simulink library "bcm"  (R2021b)
settings: Solver=VariableStepAuto  StartTime=0.0  StopTime=10.0  RelTol=1e-3
undefined symbols (not defined in the file or in its folder): ENUM_ANTITHEFT_ALARM, ENUM_ANTITHEFT_ARM, ENUM_ANTITHEFT_DISARM, ENUM_ANTITHEFT_WAIT, ENUM_GEARPOSNTOCAN_P, ENUM_PDKEYRAWLULOCK_INUNLOCK, ENUM_PDKEYRAWPS_INPS, ENUM_POWERSTA_READY, ENUM_POWERSTA_STANDBY, FALSE, KBCM_ALMBrightnessDark_enum, KBCM_AmbBlue_enum, KBCM_AmbBreathT_K, KBCM_AmbBreathTOut_K, KBCM_AmbGreen_enum, KBCM_AmbLightUser_enum, KBCM_AmbPreset_enum, KBCM_AmbRed_enum, KBCM_Antitheft_enum_ovrdflg, KBCM_Antitheft_enum_ovrdval, KBCM_APMDoorCtrlSta_flg_ovrdflg, KBCM_APMDoorCtrlSta_flg_ovrdval, KBCM_DelayTSW_flg, KBCM_DiagFLTC_mA, KBCM_DiagFMHT_s, KBCM_DiagFRTC_mA, KBCM_DiagRLTC_mA, KBCM_DiagRRTC_mA, KBCM_DrAPMRetryTimes_cnt, KBCM_DrOpenWdwOT_s, KBCM_DrOpenWdwReady_s, KBCM_ESSOffT_ms, KBCM_ESSOnT_ms, KBCM_IVIRstHoldT_ms, KBCM_IVIRstTriggerT_ms, KBCM_ONDelayT_ms, KBCM_ReDetectT_K, KBCM_RmLampKeep_min, KBCM_RmLpKeyInT_s, KBCM_RmLpKeyMissT_s, KBCM_SlpDebounceTime_s, KBCM_SPTGDetectT_sec, KBCM_SPTGLeave_flg, KBCM_SPTGLeftBound_cm, KBCM_SPTGLeftBoundOut_cm, KBCM_SPTGLowerBound_cm, KBCM_SPTGLowerBoundOut_cm, KBCM_SPTGRightBound_cm, KBCM_SPTGRightBoundOut_cm, KBCM_SPTGTOut_K, KBCM_SPTGUpperBound_cm, KBCM_SPTGUpperBoundOut_cm, KBCM_SPTGWaitDKC_sec, KBCM_USSDis_cm, KBCM_USSFilterT_K, KBCM_WaitAPMPwr_K, KBCM_WdwManualDetT_s, MIN2SEC, TRUE, XX2KXX
libraries: simulink x41, $bdroot x3, hcu_lib x2
(part 3 of 6)

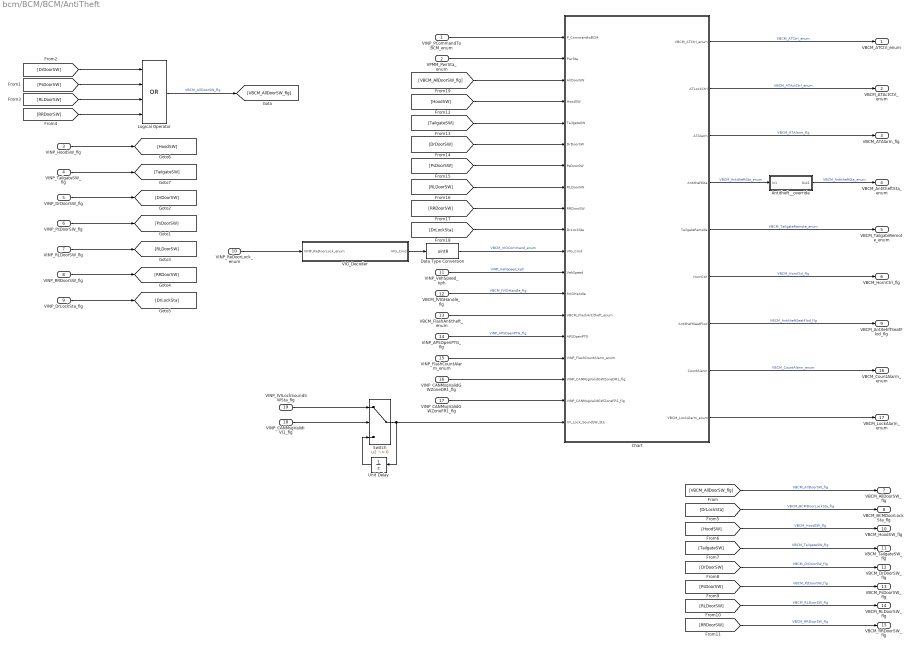
== system bcm/BCM/BCM/AntiTheft ==
  VINP_PCommandToBCM_enum : Inport
  VPMM_PwrSta_enum : Inport  Port=2
  VINP_HoodSW_flg : Inport  Port=3
  VINP_TailgateSW_flg : Inport  Port=4
  VINP_DrDoorSW_flg : Inport  Port=5
  VINP_PsDoorSW_flg : Inport  Port=6
  VINP_RLDoorSW_flg : Inport  Port=7
  VINP_RRDoorSW_flg : Inport  Port=8
  VINP_DrLockSta_flg : Inport  Port=9
  VINP_ReDoorLock_enum : Inport  Port=10
  VINP_VehSpeed_kph : Inport  Port=11
  VBCM_fVIGHandle_flg : Inport  Port=12
  VBCM_FlashAntitheft_enum : Inport  Port=13
  VINP_APSOpenPTG_flg : Inport  Port=14
  VINP_FlashCountAlarm_enum : Inport  Port=15
  VINP_CANMsgValidGWZoneDR1_flg : Inport  Port=16
  VINP_CANMsgValidGWZoneFR1_flg : Inport  Port=17
  VINP_CANMsgValidIVI1_flg : Inport  Port=18
  VINP_IVILockSoundSWSta_flg : Inport  Port=19
  Antitheft__override : Subsystem
  Chart : Stateflow chart  TreatAsAtomicUnit=on
      settings: PortSchema="{\"entries\":[{\"content\":{\"sides\":[{\"content\":{\"connectorIds\":[\"In1\",\"In2\",\"In3\",\"In4\",\"In5\",\"In6\",\"In7\",\"In8\",\"In9\",\"In10\",\"In11\",\"In12\",\"In13\",\"In14\",\"In15\",\"In16\",\"In17\",\"In18\",\"In19\"]},\"type\":\"ConnectorPlacement.EquallySpacedRectSide\",\"uuid\":\"1a74f1bb-1441-4b1e-a72b-a3afd3d564cb\"},{\"content\":{\"connectorIds\":[\"Out8\",\"Out1\",\"Out2\",\"Out3\",\"Out4\",\"Out5\",\"Out6\",\"Out7\",\"Out9\"],\"side\":\"RIGHT\"},\"type\":\"ConnectorPlacement.EquallySpacedRectSide\",\"uuid\":\"1f80d4d2-2ca7-43bd-b54c-63979ded17e1\"},{\"content\":{\"side\":\"TOP\"},\"type\":\"ConnectorPlacement.EquallySpacedRectSide\",\"uuid\":\"a2ec125f-5165-4db1-a6b4-591b84a723ff\"}]},\"type\":\"ConnectorPlacement.EquallySpacedConnector\",\"uuid\":\"5ff7fbe4-0c2a-42b5-89b8-60500b2b9a9a\"}],\"packageUris\":[\"http://schema.mathworks.com/mf0/Connector/R2020b\"],\"version\":\"1.0\"}"
  Data Type Conversion : DataTypeConversion  OutDataTypeStr=uint8
  Logical Operator : Logic  Operator=OR  Inputs=4  AllPortsSameDT=off  OutDataTypeStr=boolean
  Switch : Switch  Criteria=u2 ~= 0
  Unit Delay : UnitDelay  SampleTime=-1  HasFrameUpgradeWarning=on
  VIG_Decoder : MATLAB Function  TreatAsAtomicUnit=on
  VBCM_ATCtrl_enum : Outport
  VBCM_ATActCtrl_enum : Outport  Port=2
  VBCM_ATAlarm_flg : Outport  Port=3
  VBCM_AntitheftSta_enum : Outport  Port=4
  VBCM_TailgateRemote_enum : Outport  Port=5
  VBCM_HornCtrl_flg : Outport  Port=6
  VBCM_AllDoorSW_flg : Outport  Port=7
  VBCM_BCMDoorLockSta_flg : Outport  Port=8
  VBCM_AntitehftSeatFlod_flg : Outport  Port=9
  VBCM_HoodSW_flg : Outport  Port=10
  VBCM_TailgateSW_flg : Outport  Port=11
  VBCM_DrDoorSW_flg : Outport  Port=12
  VBCM_PsDoorSW_flg : Outport  Port=13
  VBCM_RLDoorSW_flg : Outport  Port=14
  VBCM_RRDoorSW_flg : Outport  Port=15
  VBCM_CountAlarm_enum : Outport  Port=16
  VBCM_LockAlarm_enum : Outport  Port=17
  wires:
  VBCM_fVIGHandle_flg/1 -> Chart/13(fVIGHandle)  "VBCM_fVIGHandle_flg"
  VINP_RRDoorSW_flg/1 -> [RRDoorSW]
  VINP_ReDoorLock_enum/1 -> VIG_Decoder/1(VINP_ReDoorLock_enum)
  Chart/1(ATLockCtrl) -> VBCM_ATActCtrl_enum/1  "VBCM_ATActCtrl_enum"
  Chart/8(VBCM_ATCtrl_enum) -> VBCM_ATCtrl_enum/1  "VBCM_ATCtrl_enum"
  VINP_PCommandToBCM_enum/1 -> Chart/1(P_CommandtoBCM)
  VINP_RLDoorSW_flg/1 -> [RLDoorSW]
  Chart/2(ATAlarm) -> VBCM_ATAlarm_flg/1  "VBCM_ATAlarm_flg"
  VINP_PsDoorSW_flg/1 -> [PsDoorSW]
  VINP_VehSpeed_kph/1 -> Chart/12(VehSpeed)  "VINP_VehSpeed_kph"
  Logical Operator/1 -> [VBCM_AllDoorSW_flg]  "VBCM_AllDoorSW_flg"
  VINP_DrDoorSW_flg/1 -> [DrDoorSW]
  VINP_HoodSW_flg/1 -> [HoodSW]
  VIG_Decoder/1(VIG_Cmd) -> Data Type Conversion/1
  Data Type Conversion/1 -> Chart/11(VIG_Cmd)  "VBCM_VIGCommand_enum"
  [VBCM_AllDoorSW_flg] -> VBCM_AllDoorSW_flg/1  "VBCM_AllDoorSW_flg"
  Chart/3(AntitheftSta) -> Antitheft__override/1(In1)  "VBCM_AntitheftSta_enum"
  Chart/4(TailgateRemote) -> VBCM_TailgateRemote_enum/1  "VBCM_TailgateRemote_enum"
  Chart/5(HornCtrl) -> VBCM_HornCtrl_flg/1  "VBCM_HornCtrl_flg"
  Chart/6(AntitheftSeatFlod) -> VBCM_AntitehftSeatFlod_flg/1  "VBCM_AntitheftSeatFlod_flg"
  Antitheft__override/1(Out1) -> VBCM_AntitheftSta_enum/1  "VBCM_AntitheftSta_enum"
  VINP_APSOpenPTG_flg/1 -> Chart/15(APSOpenPTG)  "VINP_APSOpenPTG_flg"
  VINP_TailgateSW_flg/1 -> [TailgateSW]
  [DrDoorSW] -> Logical Operator/1
  [PsDoorSW] -> Logical Operator/2
  [RLDoorSW] -> Logical Operator/3
  [RRDoorSW] -> Logical Operator/4
  VINP_DrLockSta_flg/1 -> [DrLockSta]
  [DrLockSta] -> VBCM_BCMDoorLockSta_flg/1  "VBCM_BCMDoorLockSta_flg"
  [HoodSW] -> VBCM_HoodSW_flg/1  "VBCM_HoodSW_flg"
  [TailgateSW] -> VBCM_TailgateSW_flg/1  "VBCM_TailgateSW_flg"
  [DrDoorSW] -> VBCM_DrDoorSW_flg/1  "VBCM_DrDoorSW_flg"
  [PsDoorSW] -> VBCM_PsDoorSW_flg/1  "VBCM_PsDoorSW_flg"
  [RLDoorSW] -> VBCM_RLDoorSW_flg/1  "VBCM_RLDoorSW_flg"
  [RRDoorSW] -> VBCM_RRDoorSW_flg/1  "VBCM_RRDoorSW_flg"
  VPMM_PwrSta_enum/1 -> Chart/2(PwrSta)
  VBCM_FlashAntitheft_enum/1 -> Chart/14(VBCM_FlashAntitheft_enum)
  [DrDoorSW] -> Chart/6(DrDoorSW)
  [TailgateSW] -> Chart/5(TailgateSW)
  [PsDoorSW] -> Chart/7(PsDoorSW)
  [HoodSW] -> Chart/4(HoodSW)
  [RRDoorSW] -> Chart/9(RRDoorSW)
  [RLDoorSW] -> Chart/8(RLDoorSW)
  [DrLockSta] -> Chart/10(DrLockSta)
  [VBCM_AllDoorSW_flg] -> Chart/3(AllDoorSW)
  VINP_FlashCountAlarm_enum/1 -> Chart/16(VINP_FlashCountAlarm_enum)
  VINP_CANMsgValidGWZoneDR1_flg/1 -> Chart/17(VINP_CANMsgValidGWZoneDR1_flg)
  VINP_CANMsgValidGWZoneFR1_flg/1 -> Chart/18(VINP_CANMsgValidGWZoneFR1_flg)
  Chart/7(CountAlarm) -> VBCM_CountAlarm_enum/1  "VBCM_CountAlarm_enum"
  Chart/9(VBCM_LockAlarm_enum) -> VBCM_LockAlarm_enum/1
  VINP_CANMsgValidIVI1_flg/1 -> Switch/2
  Unit Delay/1 -> Switch/3
  Switch/1 -> Chart/19(IVI_Lock_SoundSW_Sta), Unit Delay/1
  VINP_IVILockSoundSWSta_flg/1 -> Switch/1

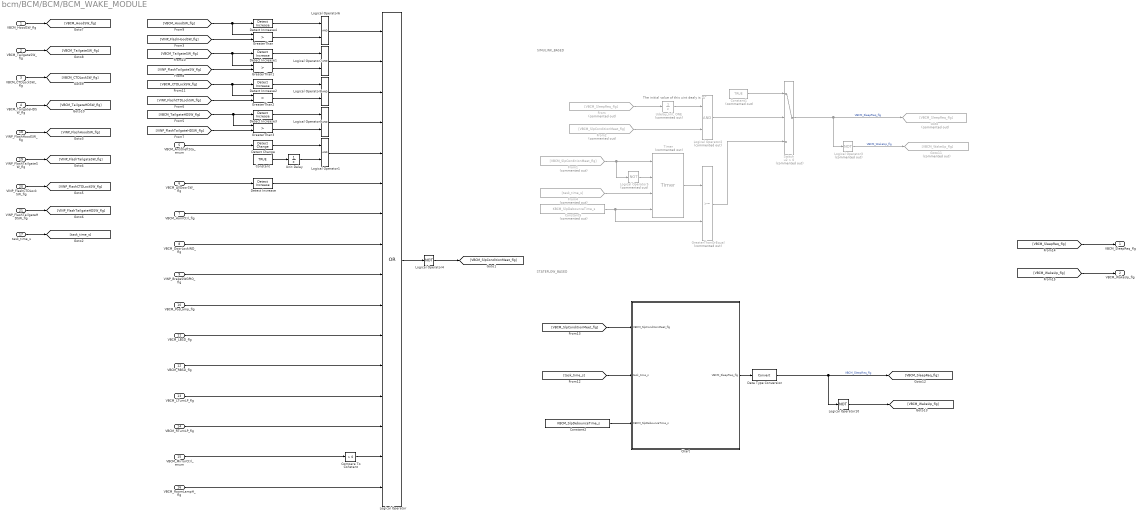
== system bcm/BCM/BCM/BCM_WAKE_MODULE ==
  note: SIMULINK_BASED
  note: STATEFLOW_BASED
  note: The initial value of this uint dealy is "1"
  VBCM_HoodSW_flg : Inport
  VBCM_TailgateSW_flg : Inport  Port=2
  VBCM_CTDLockSW_flg : Inport  Port=3
  VBCM_TailgateHDSW_flg : Inport  Port=4
  VBCM_AntitheftSta_enum : Inport  Port=5
  VBCM_AllDoorSW_flg : Inport  Port=6
  VBCM_HornCtrl_flg : Inport  Port=7
  VBCM_DoorLockIND_flg : Inport  Port=8
  VINP_BrakeSWGPIO_flg : Inport  Port=9
  VBCM_PosLamp_flg : Inport  Port=10
  VBCM_LBSD_flg : Inport  Port=11
  VBCM_RBSD_flg : Inport  Port=12
  VBCM_LTurnLP_flg : Inport  Port=13
  VBCM_RTurnLP_flg : Inport  Port=14
  VBCM_MirrorCtrl_enum : Inport  Port=15
  VBCM_RoomLampH_flg : Inport  Port=16
  task_time_s : Inport  Port=17
  VINP_FlashHoodSW_flg : Inport  Port=18
  VINP_FlashTailgateSW_flg : Inport  Port=19
  VINP_FlashCTDLockSW_flg : Inport  Port=20
  VINP_FlashTailgateHDSW_flg : Inport  Port=21
  Chart : Stateflow chart  TreatAsAtomicUnit=on
  Compare To Constant : simulink/Logic and Bit Operations/Compare To Constant  relop=>  const=0  OutDataTypeStr=boolean
  Constant : Constant  Value=TRUE
  Constant1 : Constant  Commented=on  Value=TRUE
  Constant2 : Constant  Value=KBCM_SlpDebounceTime_s
  Constant5 : Constant  Commented=on  Value=KBCM_SlpDebounceTime_s
  Data Type Conversion : DataTypeConversion
  Detect Change : simulink/Logic and Bit Operations/Detect Change  vinit=0  OutDataTypeStr=boolean
  Detect Increase{,1..4} (5 alike) : simulink/Logic and Bit Operations/Detect Increase  vinit=0.0  OutDataTypeStr=boolean
  From : From  Commented=on  GotoTag=VBCM_SleepReq_flg
  From1 : From  Commented=on  GotoTag=VBCM_SlpConditionMeet_flg
  From2 : From  Commented=on  GotoTag=VBCM_SlpConditionMeet_flg
  From4 : From  Commented=on  GotoTag=task_time_s
  Goto : Goto  Commented=on  GotoTag=VBCM_SleepReq_flg
  Goto11 : Goto  Commented=on  GotoTag=VBCM_WakeUp_flg
  GreaterThan{,1..3} (4 alike) : RelationalOperator  Operator=>  OutDataTypeStr=boolean  RndMeth=Simplest
  GreaterThanOrEqual : RelationalOperator  Commented=on  OutDataTypeStr=boolean  RndMeth=Simplest
  Logical Operator : Logic  Operator=OR  Inputs=16  AllPortsSameDT=off  OutDataTypeStr=boolean
  Logical Operator{1,6..9} (5 alike) : Logic  AllPortsSameDT=off  OutDataTypeStr=boolean
  Logical Operator10 : Logic  Operator=NOT  AllPortsSameDT=off  OutDataTypeStr=boolean
  Logical Operator2 : Logic  Commented=on  AllPortsSameDT=off  OutDataTypeStr=boolean
  Logical Operator3 : Logic  Commented=on  Operator=NOT  AllPortsSameDT=off  OutDataTypeStr=boolean
  Logical Operator4 : Logic  Operator=NOT  AllPortsSameDT=off  OutDataTypeStr=boolean
  Logical Operator5 : Logic  Commented=on  Operator=NOT  AllPortsSameDT=off  OutDataTypeStr=boolean
  Switch : Switch  Commented=on  Criteria=u2 > Threshold
  Timer : hcu_lib/Basic_Blocks/Timer  Commented=on
  Udelay_Init_ONE : UnitDelay  Commented=on  InitialCondition=1  SampleTime=-1  HasFrameUpgradeWarning=on
  Unit Delay : UnitDelay  SampleTime=-1  HasFrameUpgradeWarning=on
  VBCM_SleepReq_flg : Outport
  VBCM_WakeUp_flg : Outport  Port=2
  wires:
  VBCM_DoorLockIND_flg/1 -> Logical Operator/8
  VBCM_LBSD_flg/1 -> Logical Operator/11
  VBCM_RoomLampH_flg/1 -> Logical Operator/16
  VBCM_RBSD_flg/1 -> Logical Operator/12
  VBCM_HornCtrl_flg/1 -> Logical Operator/7
  VBCM_AllDoorSW_flg/1 -> Detect Increase/1
  VBCM_RTurnLP_flg/1 -> Logical Operator/14
  Compare To Constant/1 -> Logical Operator/15
  VBCM_PosLamp_flg/1 -> Logical Operator/10
  VINP_BrakeSWGPIO_flg/1 -> Logical Operator/9
  VBCM_MirrorCtrl_enum/1 -> Compare To Constant/1
  VBCM_LTurnLP_flg/1 -> Logical Operator/13
  Detect Change/1 -> Logical Operator1/1
  VBCM_AntitheftSta_enum/1 -> Detect Change/1
  Constant5/1 -> GreaterThanOrEqual/2, Timer/4
  Timer/1 -> GreaterThanOrEqual/1
  Logical Operator/1 -> Logical Operator4/1
  Logical Operator1/1 -> Logical Operator/5
  Unit Delay/1 -> Logical Operator1/2
  Constant/1 -> Unit Delay/1
  Logical Operator4/1 -> [VBCM_SlpConditionMeet_flg]
  Switch/1 -> Logical Operator3/1, Goto/1  "VBCM_SleepReq_flg"
  Logical Operator2/1 -> Switch/2
  Constant1/1 -> Switch/1
  From/1 -> Udelay_Init_ONE/1
  GreaterThanOrEqual/1 -> Switch/3
  Udelay_Init_ONE/1 -> Logical Operator2/1
  Logical Operator5/1 -> Timer/2
  From2/1 -> Logical Operator2/2
  From1/1 -> Logical Operator5/1, Timer/1
  task_time_s/1 -> [task_time_s]
  From4/1 -> Timer/3
  VBCM_HoodSW_flg/1 -> [VBCM_HoodSW_flg]
  [VINP_FlashHoodSW_flg] -> GreaterThan/2
  GreaterThan/1 -> Logical Operator6/2
  Logical Operator6/1 -> Logical Operator/1
  [VBCM_HoodSW_flg] -> GreaterThan/1, Detect Increase4/1
  Detect Increase4/1 -> Logical Operator6/1
  VBCM_TailgateSW_flg/1 -> [VBCM_TailgateSW_flg]
  [VBCM_CTDLockSW_flg] -> Detect Increase2/1, GreaterThan2/1
  Detect Increase2/1 -> Logical Operator8/1
  GreaterThan2/1 -> Logical Operator8/2
  Logical Operator8/1 -> Logical Operator/3
  [VINP_FlashCTDLockSW_flg] -> GreaterThan2/2
  VBCM_CTDLockSW_flg/1 -> [VBCM_CTDLockSW_flg]
  [VBCM_TailgateHDSW_flg] -> Detect Increase3/1, GreaterThan3/1
  Detect Increase3/1 -> Logical Operator9/1
  [VINP_FlashTailgateHDSW_flg] -> GreaterThan3/2
  GreaterThan3/1 -> Logical Operator9/2
  VBCM_TailgateHDSW_flg/1 -> [VBCM_TailgateHDSW_flg]
  GreaterThan1/1 -> Logical Operator7/2
  Logical Operator7/1 -> Logical Operator/2
  [VINP_FlashTailgateSW_flg] -> GreaterThan1/2
  [VBCM_TailgateSW_flg] -> GreaterThan1/1, Detect Increase1/1
  Detect Increase1/1 -> Logical Operator7/1
  Logical Operator9/1 -> Logical Operator/4
  VINP_FlashHoodSW_flg/1 -> [VINP_FlashHoodSW_flg]
  VINP_FlashTailgateSW_flg/1 -> [VINP_FlashTailgateSW_flg]
  VINP_FlashCTDLockSW_flg/1 -> [VINP_FlashCTDLockSW_flg]
  VINP_FlashTailgateHDSW_flg/1 -> [VINP_FlashTailgateHDSW_flg]
  [task_time_s] -> Chart/2(task_time_s)
  Constant2/1 -> Chart/3(KBCM_SlpDebounceTime_s)
  [VBCM_SlpConditionMeet_flg] -> Chart/1(VBCM_SlpConditionMeet_flg)
  Logical Operator3/1 -> Goto11/1  "VBCM_WakeUp_flg"
  [VBCM_SleepReq_flg] -> VBCM_SleepReq_flg/1
  [VBCM_WakeUp_flg] -> VBCM_WakeUp_flg/1
  Logical Operator10/1 -> [VBCM_WakeUp_flg]
  Data Type Conversion/1 -> Logical Operator10/1, [VBCM_SleepReq_flg]  "VBCM_SleepReq_flg"
  Chart/1(VBCM_SleepReq_flg) -> Data Type Conversion/1
  Detect Increase/1 -> Logical Operator/6

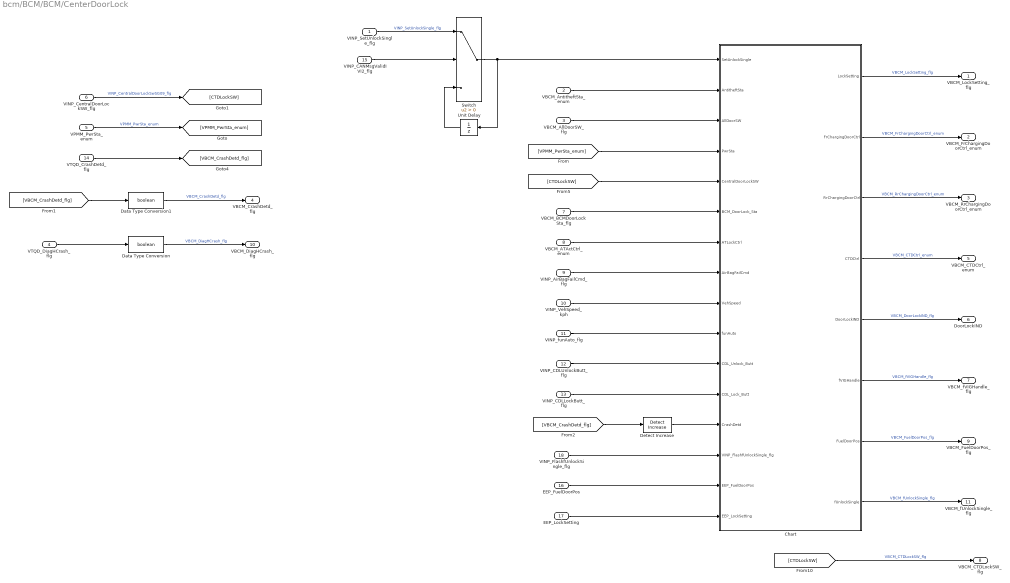
== system bcm/BCM/BCM/CenterDoorLock ==
  VINP_SetUnlockSingle_flg : Inport
  VBCM_AntitheftSta_enum : Inport  Port=2
  VBCM_AllDoorSW_flg : Inport  Port=3  OutDataTypeStr=boolean
  VTQD_DiagHCrash_flg : Inport  Port=4
  VPMM_PwrSta_enum : Inport  Port=5
  VINP_CentralDoorLockSW_flg : Inport  Port=6
  VBCM_BCMDoorLockSta_flg : Inport  Port=7
  VBCM_ATActCtrl_enum : Inport  Port=8
  VINP_AirBagFailCmd_flg : Inport  Port=9
  VINP_VehSpeed_kph : Inport  Port=10
  VINP_funAuto_flg : Inport  Port=11
  VINP_CDLUnlockButt_flg : Inport  Port=12  OutDataTypeStr=boolean
  VINP_CDLLockButt_flg : Inport  Port=13  OutDataTypeStr=boolean
  VTQD_CrashDetd_flg : Inport  Port=14
  VINP_CANMsgValidIVI2_flg : Inport  Port=15
  EEP_FuelDoorPos : Inport  Port=16
  EEP_LockSetting : Inport  Port=17
  VINP_FlashfUnlockSingle_flg : Inport  Port=18
  Chart : Stateflow chart  TreatAsAtomicUnit=on
  Data Type Conversion : DataTypeConversion  OutDataTypeStr=boolean
  Data Type Conversion1 : DataTypeConversion  OutDataTypeStr=boolean
  Detect Increase : simulink/Logic and Bit Operations/Detect Increase  vinit=0.0  OutDataTypeStr=boolean
  Switch : Switch  Criteria=u2 > Threshold
  Unit Delay : UnitDelay  SampleTime=-1  HasFrameUpgradeWarning=on
  VBCM_LockSetting_flg : Outport
  VBCM_FrChargingDoorCtrl_enum : Outport  Port=2
  VBCM_RrChargingDoorCtrl_enum : Outport  Port=3
  VBCM_CrashDetd_flg : Outport  Port=4
  VBCM_CTDCtrl_enum : Outport  Port=5
  DoorLockIND : Outport  Port=6
  VBCM_fVIGHandle_flg : Outport  Port=7
  VBCM_CTDLockSW_flg : Outport  Port=8
  VBCM_FuelDoorPos_flg : Outport  Port=9
  VBCM_DiagHCrash_flg : Outport  Port=10
  VBCM_fUnlockSingle_flg : Outport  Port=11
  wires:
  VBCM_AntitheftSta_enum/1 -> Chart/2(AntitheftSta)
  VINP_CDLUnlockButt_flg/1 -> Chart/11(CDL_Unlock_Butt)
  Chart/6(fVIGHandle) -> VBCM_fVIGHandle_flg/1  "VBCM_fVIGHandle_flg"
  Chart/1(LockSetting) -> VBCM_LockSetting_flg/1  "VBCM_LockSetting_flg"
  VINP_funAuto_flg/1 -> Chart/10(funAuto)
  VINP_VehSpeed_kph/1 -> Chart/9(VehSpeed)
  VINP_AirBagFailCmd_flg/1 -> Chart/8(AirBagFailCmd)
  VBCM_ATActCtrl_enum/1 -> Chart/7(ATLockCtrl)
  Chart/5(DoorLockIND) -> DoorLockIND/1  "VBCM_DoorLockIND_flg"
  VBCM_AllDoorSW_flg/1 -> Chart/3(AllDoorSW)
  Chart/2(FrChargingDoorCtrl) -> VBCM_FrChargingDoorCtrl_enum/1  "VBCM_FrChargingDoorCtrl_enum"
  Chart/3(RrChargingDoorCtrl) -> VBCM_RrChargingDoorCtrl_enum/1  "VBCM_RrChargingDoorCtrl_enum"
  VBCM_BCMDoorLockSta_flg/1 -> Chart/6(BCM_DoorLock_Sta)
  VINP_SetUnlockSingle_flg/1 -> Switch/1  "VINP_SetUnlockSingle_flg"
  Chart/4(CTDCtrl) -> VBCM_CTDCtrl_enum/1  "VBCM_CTDCtrl_enum"
  VINP_CDLLockButt_flg/1 -> Chart/12(CDL_Lock_Butt)
  [CTDLockSW] -> VBCM_CTDLockSW_flg/1  "VBCM_CTDLockSW_flg"
  Unit Delay/1 -> Switch/3
  Switch/1 -> Chart/1(SetUnlockSingle), Unit Delay/1
  VINP_CANMsgValidIVI2_flg/1 -> Switch/2
  VPMM_PwrSta_enum/1 -> [VPMM_PwrSta_enum]  "VPMM_PwrSta_enum"
  [VPMM_PwrSta_enum] -> Chart/4(PwrSta)
  VTQD_CrashDetd_flg/1 -> [VBCM_CrashDetd_flg]
  VINP_CentralDoorLockSW_flg/1 -> [CTDLockSW]  "VINP_CentralDoorLockSwSG09_flg"
  [CTDLockSW] -> Chart/5(CentralDoorLockSW)
  Detect Increase/1 -> Chart/13(CrashDetd)
  [VBCM_CrashDetd_flg] -> Detect Increase/1
  Data Type Conversion/1 -> VBCM_DiagHCrash_flg/1  "VBCM_DiagHCrash_flg"
  Data Type Conversion1/1 -> VBCM_CrashDetd_flg/1  "VBCM_CrashDetd_flg"
  VTQD_DiagHCrash_flg/1 -> Data Type Conversion/1
  [VBCM_CrashDetd_flg] -> Data Type Conversion1/1
  EEP_FuelDoorPos/1 -> Chart/15(EEP_FuelDoorPos)
  Chart/7(FuelDoorPos) -> VBCM_FuelDoorPos_flg/1  "VBCM_FuelDoorPos_flg"
  EEP_LockSetting/1 -> Chart/16(EEP_LockSetting)
  VINP_FlashfUnlockSingle_flg/1 -> Chart/14(VINP_FlashfUnlockSingle_flg)
  Chart/8(fUnlockSingle) -> VBCM_fUnlockSingle_flg/1  "VBCM_fUnlockSingle_flg"

== system bcm/BCM/BCM/Dimmer ==
  VINP_MFRDNBrightReq_pct : Inport
  VINP_IVIStatus_flg : Inport  Port=2
  VINP_IVINightModeSta_flg : Inport  Port=3
  VBCM_PosLamp_flag : Inport  Port=4
  VINP_CANMsgValidIVI2_flg : Inport  Port=5
  EEP_MFRDNBrightReq : Inport  Port=6
  BCMInitial : Inport  Port=7
  Chart : Stateflow chart  TreatAsAtomicUnit=on
      settings: PortSchema="{\"entries\":[{\"content\":{\"sides\":[{\"content\":{\"connectorIds\":[\"In4\",\"In1\",\"In2\",\"In3\"]},\"type\":\"ConnectorPlacement.EquallySpacedRectSide\",\"uuid\":\"076f305a-8f7e-4e65-8c9e-aa6699a69b21\"},{\"content\":{\"connectorIds\":[\"Out1\",\"Out2\"],\"side\":\"RIGHT\"},\"type\":\"ConnectorPlacement.EquallySpacedRectSide\",\"uuid\":\"bf947e95-3d60-4849-99c4-9fb941c8d282\"},{\"content\":{\"side\":\"TOP\"},\"type\":\"ConnectorPlacement.EquallySpacedRectSide\",\"uuid\":\"13c4efb7-da15-49ea-8253-a9d27aa3456c\"}]},\"type\":\"ConnectorPlacement.EquallySpacedConnector\",\"uuid\":\"7282b60f-551e-46a0-a3a5-beda89adbd0d\"}],\"packageUris\":[\"http://schema.mathworks.com/mf0/Connector/R2020b\"],\"version\":\"1.0\"}"
  Data Type Conversion1 : DataTypeConversion
  Switch1 : Switch  Criteria=u2 > Threshold
  Switch2 : Switch  Criteria=u2 > Threshold
  Switch3 : Switch  Criteria=u2 > Threshold
  Unit Delay : UnitDelay  SampleTime=-1  HasFrameUpgradeWarning=on
  Unit Delay1 : UnitDelay  SampleTime=-1  HasFrameUpgradeWarning=on
  VBCM_Dimmer_pct : Outport
  VBCM_DimmerEN_flg : Outport  Port=2
  VBCM_MFRDNBrightReq_pct : Outport  Port=3
  wires:
  VBCM_PosLamp_flag/1 -> Chart/3(PLamp)
  Chart/1(Dimmer) -> VBCM_Dimmer_pct/1  "VBCM_Dimmer_pct"
  VINP_IVIStatus_flg/1 -> Chart/1(IVI_Status)
  Chart/2(DimmerEN) -> VBCM_DimmerEN_flg/1  "VBCM_DimmerEN_flg"
  VINP_IVINightModeSta_flg/1 -> Switch1/1  "VINP_IVINightModeSta_flg"
  VINP_CANMsgValidIVI2_flg/1 -> Switch2/2, Switch1/2  "VINP_CANMsgValidIVI2_flg"
  Switch1/1 -> Unit Delay1/1, Chart/2(IVI_Night_Mode_Sta)
  Unit Delay1/1 -> Switch1/3
  BCMInitial/1 -> Switch3/2
  EEP_MFRDNBrightReq/1 -> Switch3/3
  Switch3/1 -> Data Type Conversion1/1, Unit Delay/1
  Switch2/1 -> Switch3/1
  Unit Delay/1 -> Switch2/3
  VINP_MFRDNBrightReq_pct/1 -> Switch2/1
  Data Type Conversion1/1 -> VBCM_MFRDNBrightReq_pct/1, Chart/4(MFRD_N_Bright_Req)  "VBCM_MFRDNBrightReq_pct"

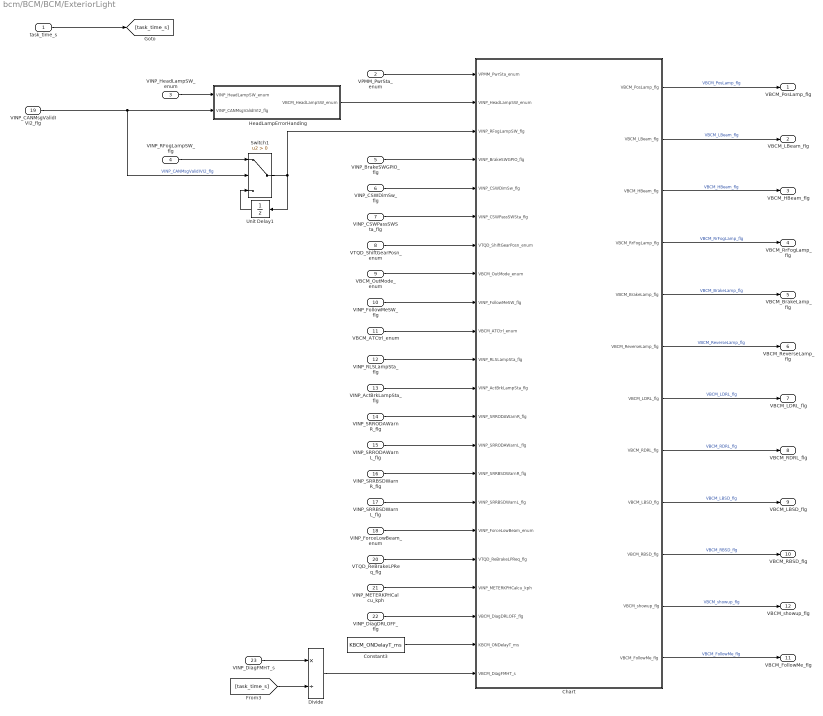
== system bcm/BCM/BCM/ExteriorLight ==
  task_time_s : Inport
  VPMM_PwrSta_enum : Inport  Port=2
  VINP_HeadLampSW_enum : Inport  Port=3
  VINP_RFogLampSW_flg : Inport  Port=4
  VINP_BrakeSWGPIO_flg : Inport  Port=5
  VINP_CSWDimSw_flg : Inport  Port=6
  VINP_CSWPassSWSta_flg : Inport  Port=7
  VTQD_ShiftGearPosn_enum : Inport  Port=8
  VBCM_OutMode_enum : Inport  Port=9
  VINP_FollowMeSW_flg : Inport  Port=10
  VBCM_ATCtrl_enum : Inport  Port=11
  VINP_RLSLampSta_flg : Inport  Port=12
  VINP_ActBrkLampSta_flg : Inport  Port=13
  VINP_SRRODAWarnR_flg : Inport  Port=14
  VINP_SRRODAWarnL_flg : Inport  Port=15
  VINP_SRRBSDWarnR_flg : Inport  Port=16
  VINP_SRRBSDWarnL_flg : Inport  Port=17
  VINP_ForceLowBeam_enum : Inport  Port=18
  VINP_CANMsgValidIVI2_flg : Inport  Port=19
  VTQD_ReBrakeLPReq_flg : Inport  Port=20
  VINP_METERKPHCalcu_kph : Inport  Port=21
  VINP_DiagDRLOFF_flg : Inport  Port=22
  VINP_DiagFMHT_s : Inport  Port=23
  Chart : Stateflow chart  TreatAsAtomicUnit=on
      settings: PortSchema="{\"entries\":[{\"content\":{\"sides\":[{\"content\":{\"connectorIds\":[\"In1\",\"In2\",\"In3\",\"In4\",\"In5\",\"In6\",\"In7\",\"In8\",\"In9\",\"In10\",\"In11\",\"In12\",\"In13\",\"In14\",\"In15\",\"In16\",\"In17\",\"In18\",\"In21\",\"In19\",\"In22\",\"In20\"]},\"type\":\"ConnectorPlacement.EquallySpacedRectSide\",\"uuid\":\"34a74b70-26ca-4365-9514-cef344c89284\"},{\"content\":{\"connectorIds\":[\"Out1\",\"Out2\",\"Out3\",\"Out4\",\"Out5\",\"Out6\",\"Out7\",\"Out8\",\"Out9\",\"Out10\",\"Out11\",\"Out12\"],\"side\":\"RIGHT\"},\"type\":\"ConnectorPlacement.EquallySpacedRectSide\",\"uuid\":\"35b33564-17af-4a68-ba31-40ca81daf0a6\"},{\"content\":{\"connectorIds\":[],\"side\":\"TOP\"},\"type\":\"ConnectorPlacement.EquallySpacedRectSide\",\"uuid\":\"ba3f7f15-bc53-4e23-8d24-280f07cf706f\"}]},\"type\":\"ConnectorPlacement.EquallySpacedConnector\",\"uuid\":\"116adca9-6a34-4fe6-9115-066bd056288e\"}],\"packageUris\":[\"http://schema.mathworks.com/mf0/Connector/R2020b\"],\"version\":\"1.0\"}"
  Constant3 : Constant  Value=KBCM_ONDelayT_ms
  Divide : Product  Inputs=*/
  HeadLampErrorHanding : Subsystem
  Switch1 : Switch  Criteria=u2 > Threshold
  Unit Delay1 : UnitDelay  SampleTime=-1  HasFrameUpgradeWarning=on
  VBCM_PosLamp_flg : Outport
  VBCM_LBeam_flg : Outport  Port=2
  VBCM_HBeam_flg : Outport  Port=3
  VBCM_RrFogLamp_flg : Outport  Port=4
  VBCM_BrakeLamp_flg : Outport  Port=5
  VBCM_ReverseLamp_flg : Outport  Port=6
  VBCM_LDRL_flg : Outport  Port=7
  VBCM_RDRL_flg : Outport  Port=8
  VBCM_LBSD_flg : Outport  Port=9
  VBCM_RBSD_flg : Outport  Port=10
  VBCM_FollowMe_flg : Outport  Port=11
  VBCM_showup_flg : Outport  Port=12
  wires:
  Chart/11(VBCM_showup_flg) -> VBCM_showup_flg/1  "VBCM_showup_flg"
  VTQD_ReBrakeLPReq_flg/1 -> Chart/18(VTQD_ReBrakeLPReq_flg)
  VINP_DiagDRLOFF_flg/1 -> Chart/19(VBCM_DiagDRLOFF_flg)
  Unit Delay1/1 -> Switch1/3
  VINP_CANMsgValidIVI2_flg/1 -> Switch1/2, HeadLampErrorHanding/2(VINP_CANMsgValidIVI2_flg)  "VINP_CANMsgValidIVI2_flg"
  Switch1/1 -> Chart/3(VINP_RFogLampSW_flg), Unit Delay1/1
  Chart/6(VBCM_ReverseLamp_flg) -> VBCM_ReverseLamp_flg/1  "VBCM_ReverseLamp_flg"
  VTQD_ShiftGearPosn_enum/1 -> Chart/7(VTQD_ShiftGearPosn_enum)
  VINP_CSWDimSw_flg/1 -> Chart/5(VINP_CSWDimSw_flg)
  VBCM_ATCtrl_enum/1 -> Chart/10(VBCM_ATCtrl_enum)
  Chart/9(VBCM_LBSD_flg) -> VBCM_LBSD_flg/1  "VBCM_LBSD_flg"
  VINP_RLSLampSta_flg/1 -> Chart/11(VINP_RLSLampSta_flg)
  VINP_SRRBSDWarnR_flg/1 -> Chart/15(VINP_SRRBSDWarnR_flg)
  VINP_SRRBSDWarnL_flg/1 -> Chart/16(VINP_SRRBSDWarnL_flg)
  VINP_ActBrkLampSta_flg/1 -> Chart/12(VINP_ActBrkLampSta_flg)
  VINP_SRRODAWarnL_flg/1 -> Chart/14(VINP_SRRODAWarnL_flg)
  VINP_FollowMeSW_flg/1 -> Chart/9(VINP_FollowMeSW_flg)
  VINP_ForceLowBeam_enum/1 -> Chart/17(VINP_ForceLowBeam_enum)
  VINP_SRRODAWarnR_flg/1 -> Chart/13(VINP_SRRODAWarnR_flg)
  Chart/10(VBCM_RBSD_flg) -> VBCM_RBSD_flg/1  "VBCM_RBSD_flg"
  VBCM_OutMode_enum/1 -> Chart/8(VBCM_OutMode_enum)
  VINP_BrakeSWGPIO_flg/1 -> Chart/4(VINP_BrakeSWGPIO_flg)
  VINP_CSWPassSWSta_flg/1 -> Chart/6(VINP_CSWPassSWSta_flg)
  Chart/3(VBCM_HBeam_flg) -> VBCM_HBeam_flg/1  "VBCM_HBeam_flg"
  Chart/4(VBCM_RrFogLamp_flg) -> VBCM_RrFogLamp_flg/1  "VBCM_RrFogLamp_flg"
  VINP_RFogLampSW_flg/1 -> Switch1/1
  Chart/5(VBCM_BrakeLamp_flg) -> VBCM_BrakeLamp_flg/1  "VBCM_BrakeLamp_flg"
  Chart/2(VBCM_LBeam_flg) -> VBCM_LBeam_flg/1  "VBCM_LBeam_flg"
  Chart/7(VBCM_LDRL_flg) -> VBCM_LDRL_flg/1  "VBCM_LDRL_flg"
  Chart/8(VBCM_RDRL_flg) -> VBCM_RDRL_flg/1  "VBCM_RDRL_flg"
  VPMM_PwrSta_enum/1 -> Chart/1(VPMM_PwrSta_enum)
  Chart/1(VBCM_PosLamp_flg) -> VBCM_PosLamp_flg/1  "VBCM_PosLamp_flg"
  VINP_METERKPHCalcu_kph/1 -> Chart/21(VINP_METERKPHCalcu_kph)
  Constant3/1 -> Chart/22(KBCM_ONDelayT_ms)
  VINP_HeadLampSW_enum/1 -> HeadLampErrorHanding/1(VINP_HeadLampSW_enum)
  HeadLampErrorHanding/1(VBCM_HeadLampSW_enum) -> Chart/2(VINP_HeadLampSW_enum)
  Chart/12(VBCM_FollowMe_flg) -> VBCM_FollowMe_flg/1  "VBCM_FollowMe_flg"
  [task_time_s] -> Divide/2
  Divide/1 -> Chart/20(VBCM_DiagFMHT_s)
  task_time_s/1 -> [task_time_s]
  VINP_DiagFMHT_s/1 -> Divide/1

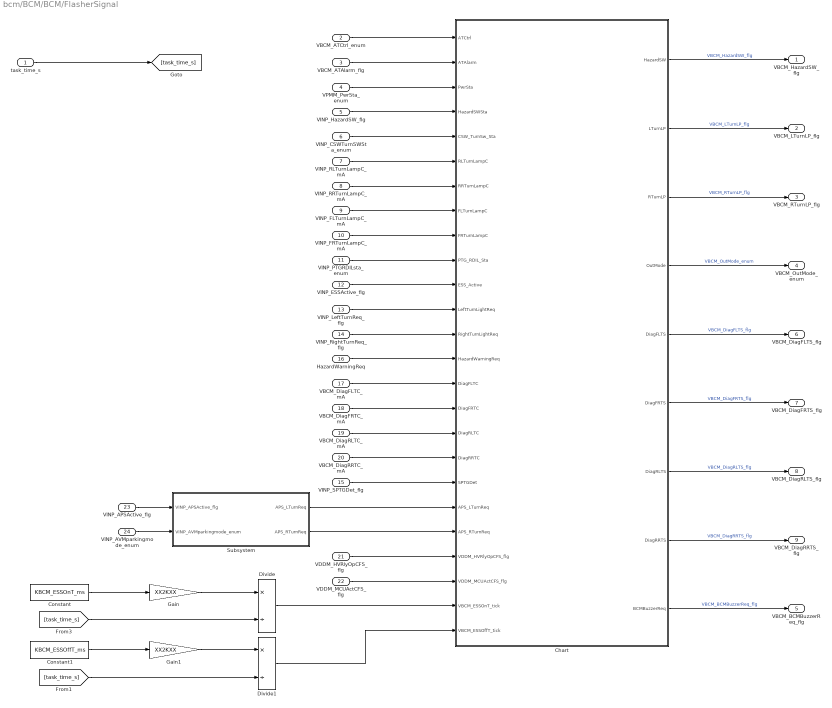
== system bcm/BCM/BCM/FlasherSignal ==
  task_time_s : Inport
  VBCM_ATCtrl_enum : Inport  Port=2
  VBCM_ATAlarm_flg : Inport  Port=3
  VPMM_PwrSta_enum : Inport  Port=4
  VINP_HazardSW_flg : Inport  Port=5
  VINP_CSWTurnSWSta_enum : Inport  Port=6
  VINP_RLTurnLampC_mA : Inport  Port=7
  VINP_RRTurnLampC_mA : Inport  Port=8
  VINP_FLTurnLampC_mA : Inport  Port=9
  VINP_FRTurnLampC_mA : Inport  Port=10
  VINP_PTGRDILsta_enum : Inport  Port=11
  VINP_ESSActive_flg : Inport  Port=12
  VINP_LeftTurnReq_flg : Inport  Port=13
  VINP_RightTurnReq_flg : Inport  Port=14
  VINP_SPTGDet_flg : Inport  Port=15
  HazardWarningReq : Inport  Port=16
  VBCM_DiagFLTC_mA : Inport  Port=17
  VBCM_DiagFRTC_mA : Inport  Port=18
  VBCM_DiagRLTC_mA : Inport  Port=19
  VBCM_DiagRRTC_mA : Inport  Port=20
  VDDM_HVRlyOpCFS_flg : Inport  Port=21
  VDDM_MCUActCFS_flg : Inport  Port=22
  VINP_APSActive_flg : Inport  Port=23
  VINP_AVMparkingmode_enum : Inport  Port=24
  Chart : Stateflow chart  TreatAsAtomicUnit=on
      settings: PortSchema="{\"entries\":[{\"content\":{\"sides\":[{\"content\":{\"connectorIds\":[\"In1\",\"In2\",\"In3\",\"In4\",\"In5\",\"In6\",\"In7\",\"In8\",\"In9\",\"In10\",\"In11\",\"In12\",\"In13\",\"In15\",\"In16\",\"In17\",\"In18\",\"In19\",\"In14\",\"In20\",\"In21\",\"In22\",\"In23\",\"In25\",\"In24\"]},\"type\":\"ConnectorPlacement.EquallySpacedRectSide\",\"uuid\":\"fb222101-3ebe-4085-bdf3-20ef70df8d28\"},{\"content\":{\"connectorIds\":[\"Out1\",\"Out2\",\"Out3\",\"Out4\",\"Out5\",\"Out6\",\"Out7\",\"Out8\",\"Out9\"],\"side\":\"RIGHT\"},\"type\":\"ConnectorPlacement.EquallySpacedRectSide\",\"uuid\":\"1d165777-adb5-42aa-9b79-2429bdff6c1c\"},{\"content\":{\"connectorIds\":[],\"side\":\"TOP\"},\"type\":\"ConnectorPlacement.EquallySpacedRectSide\",\"uuid\":\"46eb436b-9b3b-4f68-9e11-94686797b079\"}]},\"type\":\"ConnectorPlacement.EquallySpacedConnector\",\"uuid\":\"ccb97afc-e3e1-4b58-940d-fbdbd7472620\"}],\"packageUris\":[\"http://schema.mathworks.com/mf0/Connector/R2020b\"],\"version\":\"1.0\"}"
  Constant : Constant  Value=KBCM_ESSOnT_ms
  Constant1 : Constant  Value=KBCM_ESSOffT_ms
  Divide : Product  Inputs=*/
  Divide1 : Product  Inputs=*/
  Gain : Gain  Gain=XX2KXX
  Gain1 : Gain  Gain=XX2KXX
  Subsystem : Subsystem
  VBCM_HazardSW_flg : Outport
  VBCM_LTurnLP_flg : Outport  Port=2
  VBCM_RTurnLP_flg : Outport  Port=3
  VBCM_OutMode_enum : Outport  Port=4
  VBCM_BCMBuzzerReq_flg : Outport  Port=5
  VBCM_DiagFLTS_flg : Outport  Port=6
  VBCM_DiagFRTS_flg : Outport  Port=7
  VBCM_DiagRLTS_flg : Outport  Port=8
  VBCM_DiagRRTS_flg : Outport  Port=9
  wires:
  Chart/1(HazardSW) -> VBCM_HazardSW_flg/1  "VBCM_HazardSW_flg"
  VINP_RRTurnLampC_mA/1 -> Chart/7(RRTurnLampC)
  Chart/3(RTurnLP) -> VBCM_RTurnLP_flg/1  "VBCM_RTurnLP_flg"
  VBCM_ATCtrl_enum/1 -> Chart/1(ATCtrl)
  Chart/2(LTurnLP) -> VBCM_LTurnLP_flg/1  "VBCM_LTurnLP_flg"
  VINP_RLTurnLampC_mA/1 -> Chart/6(RLTurnLampC)
  VPMM_PwrSta_enum/1 -> Chart/3(PwrSta)
  VINP_HazardSW_flg/1 -> Chart/4(HazardSWSta)
  VINP_FRTurnLampC_mA/1 -> Chart/9(FRTurnLampC)
  Chart/4(OutMode) -> VBCM_OutMode_enum/1  "VBCM_OutMode_enum"
  VBCM_ATAlarm_flg/1 -> Chart/2(ATAlarm)
  VINP_FLTurnLampC_mA/1 -> Chart/8(FLTurnLampC)
  VINP_CSWTurnSWSta_enum/1 -> Chart/5(CSW_TurnSw_Sta)
  VINP_ESSActive_flg/1 -> Chart/11(ESS_Active)
  VINP_LeftTurnReq_flg/1 -> Chart/12(LeftTurnLightReq)
  VINP_RightTurnReq_flg/1 -> Chart/13(RightTurnLightReq)
  VINP_PTGRDILsta_enum/1 -> Chart/10(PTG_RDIL_Sta)
  HazardWarningReq/1 -> Chart/15(HazardWarningReq)
  VINP_SPTGDet_flg/1 -> Chart/14(SPTGDet)
  Chart/9(BCMBuzzerReq) -> VBCM_BCMBuzzerReq_flg/1  "VBCM_BCMBuzzerReq_flg"
  VDDM_HVRlyOpCFS_flg/1 -> Chart/22(VDDM_HVRlyOpCFS_flg)
  VDDM_MCUActCFS_flg/1 -> Chart/23(VDDM_MCUActCFS_flg)
  Chart/6(DiagFRTS) -> VBCM_DiagFRTS_flg/1  "VBCM_DiagFRTS_flg"
  Chart/7(DiagRLTS) -> VBCM_DiagRLTS_flg/1  "VBCM_DiagRLTS_flg"
  Chart/5(DiagFLTS) -> VBCM_DiagFLTS_flg/1  "VBCM_DiagFLTS_flg"
  Chart/8(DiagRRTS) -> VBCM_DiagRRTS_flg/1  "VBCM_DiagRRTS_flg"
  VINP_APSActive_flg/1 -> Subsystem/1(VINP_APSActive_flg)
  VINP_AVMparkingmode_enum/1 -> Subsystem/2(VINP_AVMparkingmode_enum)
  Subsystem/1(APS_LTurnReq) -> Chart/20(APS_LTurnReq)
  Subsystem/2(APS_RTurnReq) -> Chart/21(APS_RTurnReq)
  VBCM_DiagFLTC_mA/1 -> Chart/16(DiagFLTC)
  VBCM_DiagFRTC_mA/1 -> Chart/17(DiagFRTC)
  VBCM_DiagRLTC_mA/1 -> Chart/18(DiagRLTC)
  VBCM_DiagRRTC_mA/1 -> Chart/19(DiagRRTC)
  [task_time_s] -> Divide/2
  Gain/1 -> Divide/1
  Constant/1 -> Gain/1
  task_time_s/1 -> [task_time_s]
  Constant1/1 -> Gain1/1
  Gain1/1 -> Divide1/1
  [task_time_s] -> Divide1/2
  Divide/1 -> Chart/25(VBCM_ESSOnT_tick)
  Divide1/1 -> Chart/24(VBCM_ESSOffT_tick)

== system bcm/BCM/BCM/IVI Reset ==
  VINP_SWCmodeSta_flg : Inport
  KBCM_IVIRstHoldT_ms : Inport  Port=2
  KBCM_IVIRstTriggerT_ms : Inport  Port=3
  Chart : Stateflow chart  TreatAsAtomicUnit=on
      settings: PortSchema="{\"entries\":[{\"content\":{\"sides\":[{\"content\":{\"connectorIds\":[\"In3\",\"In1\",\"In2\"]},\"type\":\"ConnectorPlacement.EquallySpacedRectSide\",\"uuid\":\"527c4af8-44de-47f2-8701-d5f5b7b571d6\"},{\"content\":{\"connectorIds\":[\"Out1\"],\"side\":\"RIGHT\"},\"type\":\"ConnectorPlacement.EquallySpacedRectSide\",\"uuid\":\"5335a623-2c87-4967-8624-b1c657e6893f\"},{\"content\":{\"connectorIds\":[],\"side\":\"TOP\"},\"type\":\"ConnectorPlacement.EquallySpacedRectSide\",\"uuid\":\"ed42b152-df02-4687-bffb-78347cddc5c0\"}]},\"type\":\"ConnectorPlacement.EquallySpacedConnector\",\"uuid\":\"716ba71d-aae5-4637-96c7-fec6e8a69169\"}],\"packageUris\":[\"http://schema.mathworks.com/mf0/Connector/R2020b\"],\"version\":\"1.0\"}"
  Gain : Gain  Gain=1/10
  Gain1 : Gain  Gain=1/10
  Ground : Ground
  Terminator : Terminator
  VBCM_IVIRST_flg : Outport
  wires:
  KBCM_IVIRstHoldT_ms/1 -> Gain/1
  KBCM_IVIRstTriggerT_ms/1 -> Gain1/1
  VINP_SWCmodeSta_flg/1 -> Chart/3(VINP_SWCmodeSta_flg)
  Gain/1 -> Chart/1(KBCM_IVIRstHoldT_ms)
  Gain1/1 -> Chart/2(KBCM_IVIRstTriggerT_ms)
  Chart/1(VBCM_IVIRST_flg) -> Terminator/1
  Ground/1 -> VBCM_IVIRST_flg/1  "VBCM_IVIRST_flg"

== system bcm/BCM/BCM/PTG ==
  VINP_PDKeyAreaPTG_enum : Inport
  VINP_TailgateSW_flg : Inport  Port=2
  VAPM_PASDRMR_cm : Inport  Port=3
  VAPM_PASDRML_cm : Inport  Port=4
  VINP_PCommandToBCM_enum : Inport  Port=5
  VPMM_PwrSta_eunm : Inport  Port=6
  VTQD_ShiftGearPosn_enum : Inport  Port=7
  VINP_IVIPTGUSStaSW_flg : Inport  Port=8
  VINP_CANMsgValidIVI2_flg : Inport  Port=9
  VINP_VehSpeed_kph : Inport  Port=10
  VINP_CANMsgValidDKC1_flg : Inport  Port=11
  KBCM_DelayTSW_flg : Inport  Port=12
  KBCM_ReDetectT_K : Inport  Port=13
  KBCM_SPTGDetectT_sec : Inport  Port=14
  KBCM_SPTGLeave_flg : Inport  Port=15
  KBCM_SPTGWaitDKC_sec : Inport  Port=16
  EEP_IVIPTGUSStaSW : Inport  Port=17
  BCMInitial : Inport  Port=18
  Chart : Stateflow chart  TreatAsAtomicUnit=on
      settings: PortSchema="{\"entries\":[{\"content\":{\"sides\":[{\"content\":{\"connectorIds\":[\"In1\",\"In13\",\"In14\",\"In15\",\"In16\",\"In3\",\"In2\",\"In7\",\"In4\",\"In5\",\"In6\",\"In8\",\"In9\",\"In10\",\"In11\",\"In12\"]},\"type\":\"ConnectorPlacement.EquallySpacedRectSide\",\"uuid\":\"2c0d242d-6a76-4137-8e1d-4d6809bc83cf\"},{\"content\":{\"connectorIds\":[\"Out2\",\"Out1\"],\"side\":\"RIGHT\"},\"type\":\"ConnectorPlacement.EquallySpacedRectSide\",\"uuid\":\"af4f90f4-f68e-4fa9-bb59-784446720a84\"},{\"content\":{\"side\":\"TOP\"},\"type\":\"ConnectorPlacement.EquallySpacedRectSide\",\"uuid\":\"f397bac8-7d09-437c-83a0-3821a6ac718f\"}]},\"type\":\"ConnectorPlacement.EquallySpacedConnector\",\"uuid\":\"a750c59f-e2db-4dfa-b2ae-496db5c88784\"}],\"packageUris\":[\"http://schema.mathworks.com/mf0/Connector/R2020b\"],\"version\":\"1.0\"}"
  Compare To Constant : simulink/Logic and Bit Operations/Compare To Constant  relop===  const=1  OutDataTypeStr=boolean
  Detect Change : simulink/Logic and Bit Operations/Detect Change  vinit=0  OutDataTypeStr=boolean
  KeyDetected : Subsystem
  Subsystem1 : Subsystem
  Subsystem3 : Subsystem
  Switch : Switch  Criteria=u2 > Threshold
  Switch2 : Switch  Criteria=u2 > Threshold
  Switch3 : Switch  Criteria=u2 > Threshold
  Unit Delay1 : UnitDelay  SampleTime=-1  HasFrameUpgradeWarning=on
  Unit Delay2 : UnitDelay  SampleTime=-1  HasFrameUpgradeWarning=on
  VBCM_SPTGDet_flg : Outport
  VBCM_APSOpenPTG_flg : Outport  Port=2
  VBCM_IVIPTGUSStaSW_flg : Outport  Port=3
  wires:
  KeyDetected/1(KeyDetected) -> Chart/2(KeyDetected)  "VBCM_PASKeyDetected_flg"
  VINP_VehSpeed_kph/1 -> Chart/9(VehSpeed)
  VINP_PCommandToBCM_enum/1 -> Detect Change/1
  VTQD_ShiftGearPosn_enum/1 -> Chart/11(ShiftGearPosn)
  VINP_TailgateSW_flg/1 -> Chart/8(TailgateSW)
  Chart/1(VBCM_APSOpenPTG_flg) -> VBCM_APSOpenPTG_flg/1
  Detect Change/1 -> Chart/10(DKCKeyPress)  "DKCKeyPress"
  VPMM_PwrSta_eunm/1 -> Chart/6(PwrSta)
  Chart/2(VBCM_SPTGDet_flg) -> VBCM_SPTGDet_flg/1
  KBCM_DelayTSW_flg/1 -> Chart/1(KBCM_DelayTSW_flg)
  Subsystem1/1(PASDRMR) -> KeyDetected/1(VBCM_PASDRMR_cm), Chart/3(PASDRMR)  "VBCM_PASDRMRF_cm"
  Subsystem3/1(PASDRML) -> Chart/4(PASDRML), KeyDetected/2(VBCM_PASDRML_cm)  "VBCM_PASDRMLF_cm"
  KBCM_ReDetectT_K/1 -> Chart/13(KBCM_ReDetectT_K)
  VAPM_PASDRMR_cm/1 -> Subsystem1/1(VAPM_PASDRMR_cm)
  VAPM_PASDRML_cm/1 -> Subsystem3/1(VAPM_PASDRML_cm)
  Switch/1 -> Unit Delay1/1, Compare To Constant/1
  Unit Delay1/1 -> Switch/3
  VINP_PDKeyAreaPTG_enum/1 -> Switch/1
  VINP_CANMsgValidDKC1_flg/1 -> Switch/2
  KBCM_SPTGDetectT_sec/1 -> Chart/14(KBCM_SPTGDetectT_sec)
  KeyDetected/2(KeyDetectedOut) -> Chart/7(KeyDetectedOut)
  KBCM_SPTGLeave_flg/1 -> Chart/15(KBCM_SPTGLeave_flg)
  Compare To Constant/1 -> Chart/5(PDKeyAreaPTG)
  KBCM_SPTGWaitDKC_sec/1 -> Chart/16(KBCM_SPTGWaitDKC_sec)
  Unit Delay2/1 -> Switch2/3
  VINP_IVIPTGUSStaSW_flg/1 -> Switch2/1
  VINP_CANMsgValidIVI2_flg/1 -> Switch2/2  "VINP_CANMsgValidIVI2_flg"
  EEP_IVIPTGUSStaSW/1 -> Switch3/3
  Switch2/1 -> Switch3/1
  BCMInitial/1 -> Switch3/2
  Switch3/1 -> VBCM_IVIPTGUSStaSW_flg/1, Unit Delay2/1, Chart/12(IVI_PTG_USSta_SW)  "VBCM_IVIPTGUSStaSW_flg"

== system bcm/BCM/BCM/PowerMirror ==
  VPMM_PwrSta_enum : Inport
  VINP_MIRRORFOLDSW_flg : Inport  Port=2
  VINP_VehSpeed_kph : Inport  Port=3
  VBCM_ATActCtrl_enum : Inport  Port=4
  VINP_ReOutsideMirror_enum : Inport  Port=5
  EEP_MFSWTri_flg : Inport  Port=6
  EEP_MirrorFlodPos : Inport  Port=7
  Chart : Stateflow chart  TreatAsAtomicUnit=on
  VBCM_MirrorCtrl_enum : Outport
  MFSWTri : Outport  Port=2
  MirrorFlodPos : Outport  Port=3
  wires:
  VPMM_PwrSta_enum/1 -> Chart/1(PwrSta)
  VINP_MIRRORFOLDSW_flg/1 -> Chart/2(MirrorFoldSw)
  Chart/1(MirrorCtrl) -> VBCM_MirrorCtrl_enum/1  "VBCM_MirrorCtrl_enum"
  VBCM_ATActCtrl_enum/1 -> Chart/4(ATActCtrl)
  VINP_VehSpeed_kph/1 -> Chart/3(VehSpeed)
  VINP_ReOutsideMirror_enum/1 -> Chart/5(VINP_ReOutsideMirror_enum)
  EEP_MFSWTri_flg/1 -> Chart/6(EEP_MFSWTri_flg)
  EEP_MirrorFlodPos/1 -> Chart/7(EEP_MirrorFlodPos)
  Chart/2(MFSWTri) -> MFSWTri/1  "VBCM_MFSWTri_flg"
  Chart/3(MirrorFlodPos) -> MirrorFlodPos/1  "VBCM_MirrorFlodPos_flg"

== system bcm/BCM/BCM/RearDefogger ==
  VPMM_PwrSta_enum : Inport
  VINP_RRDefSta_flg : Inport  Port=2
  VINP_IVIRRDefReq_flg : Inport  Port=3
  Chart : Stateflow chart  TreatAsAtomicUnit=on
  VBCM_MirrorDefog_flg : Outport
  VBCM_RrDefog_flg : Outport  Port=2
  wires:
  Chart/1(MirrorDefog) -> VBCM_MirrorDefog_flg/1  "VBCM_MirrorDefog_flg"
  VINP_IVIRRDefReq_flg/1 -> Chart/3(IVI_RR_Def_Req)
  VPMM_PwrSta_enum/1 -> Chart/1(PwrSta)
  Chart/2(RearDefog) -> VBCM_RrDefog_flg/1  "VBCM_RrDefog_flg"
  VINP_RRDefSta_flg/1 -> Chart/2(RR_Def_Sta)

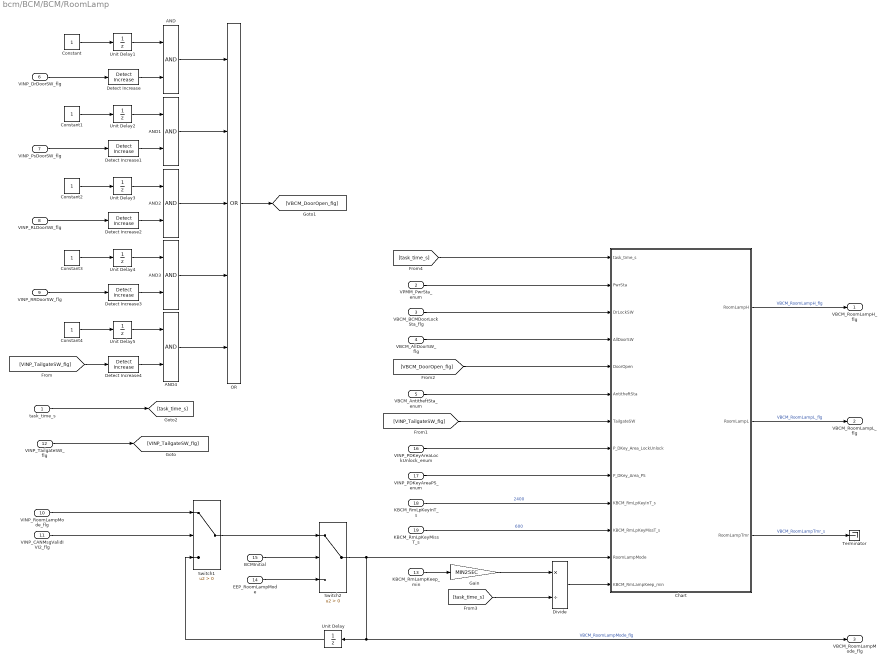
== system bcm/BCM/BCM/RoomLamp ==
  task_time_s : Inport
  VPMM_PwrSta_enum : Inport  Port=2
  VBCM_BCMDoorLockSta_flg : Inport  Port=3
  VBCM_AllDoorSW_flg : Inport  Port=4
  VBCM_AntitheftSta_enum : Inport  Port=5
  VINP_DrDoorSW_flg : Inport  Port=6
  VINP_PsDoorSW_flg : Inport  Port=7
  VINP_RLDoorSW_flg : Inport  Port=8
  VINP_RRDoorSW_flg : Inport  Port=9
  VINP_RoomLampMode_flg : Inport  Port=10
  VINP_CANMsgValidIVI2_flg : Inport  Port=11
  VINP_TailgateSW_flg : Inport  Port=12
  KBCM_RmLampKeep_min : Inport  Port=13
  EEP_RoomLampMode : Inport  Port=14
  BCMInitial : Inport  Port=15
  VINP_PDKeyAreaLockUnlock_enum : Inport  Port=16
  VINP_PDKeyAreaPS_enum : Inport  Port=17
  KBCM_RmLpKeyInT_s : Inport  Port=18
  KBCM_RmLpKeyMissT_s : Inport  Port=19
  AND{,1..4} (5 alike) : Logic  AllPortsSameDT=off  OutDataTypeStr=boolean
  Chart : Stateflow chart  TreatAsAtomicUnit=on
      settings: PortSchema="{\"entries\":[{\"content\":{\"sides\":[{\"content\":{\"connectorIds\":[\"In1\",\"In2\",\"In3\",\"In4\",\"In5\",\"In6\",\"In7\",\"In10\",\"In11\",\"In12\",\"In13\",\"In9\",\"In8\"]},\"type\":\"ConnectorPlacement.EquallySpacedRectSide\",\"uuid\":\"6d4ef6e4-d310-4573-8670-c3ce7ffc5586\"},{\"content\":{\"connectorIds\":[\"Out1\",\"Out2\",\"Out3\"],\"side\":\"RIGHT\"},\"type\":\"ConnectorPlacement.EquallySpacedRectSide\",\"uuid\":\"4b29c1e1-9016-4f15-a64e-722acfc91947\"},{\"content\":{\"connectorIds\":[],\"side\":\"TOP\"},\"type\":\"ConnectorPlacement.EquallySpacedRectSide\",\"uuid\":\"c4982b23-9105-4f8b-8d41-99f0f59e85fc\"}]},\"type\":\"ConnectorPlacement.EquallySpacedConnector\",\"uuid\":\"68c6e652-9227-465e-b41e-a009e64da19a\"}],\"packageUris\":[\"http://schema.mathworks.com/mf0/Connector/R2020b\"],\"version\":\"1.0\"}"
  Constant{,1..4} (5 alike) : Constant  OutDataTypeStr=uint8
  Detect Increase{,1..4} (5 alike) : simulink/Logic and Bit Operations/Detect Increase  vinit=0.0  OutDataTypeStr=boolean
  Divide : Product  Inputs=*/
  Gain : Gain  Gain=MIN2SEC
  OR : Logic  Operator=OR  Inputs=5  AllPortsSameDT=off  OutDataTypeStr=boolean
  Switch1 : Switch  Criteria=u2 > Threshold
  Switch2 : Switch  Criteria=u2 > Threshold
  Terminator : Terminator
  Unit Delay{,1..5} (6 alike) : UnitDelay  SampleTime=-1  HasFrameUpgradeWarning=on
  VBCM_RoomLampH_flg : Outport
  VBCM_RoomLampL_flg : Outport  Port=2
  VBCM_RoomLampMode_flg : Outport  Port=3
  wires:
  VBCM_BCMDoorLockSta_flg/1 -> Chart/3(DrLockSW)
  Chart/2(RoomLampL) -> VBCM_RoomLampL_flg/1  "VBCM_RoomLampL_flg"
  VPMM_PwrSta_enum/1 -> Chart/2(PwrSta)
  VBCM_AllDoorSW_flg/1 -> Chart/4(AllDoorSW)
  Chart/1(RoomLampH) -> VBCM_RoomLampH_flg/1  "VBCM_RoomLampH_flg"
  VBCM_AntitheftSta_enum/1 -> Chart/6(AntitheftSta)
  KBCM_RmLampKeep_min/1 -> Gain/1
  Gain/1 -> Divide/1
  Switch1/1 -> Switch2/1
  VINP_CANMsgValidIVI2_flg/1 -> Switch1/2
  Unit Delay/1 -> Switch1/3
  Switch2/1 -> VBCM_RoomLampMode_flg/1, Unit Delay/1, Chart/9(RoomLampMode)  "VBCM_RoomLampMode_flg"
  VINP_RoomLampMode_flg/1 -> Switch1/1
  BCMInitial/1 -> Switch2/2
  EEP_RoomLampMode/1 -> Switch2/3
  Constant/1 -> Unit Delay1/1
  Unit Delay1/1 -> AND/1
  Detect Increase/1 -> AND/2
  VINP_DrDoorSW_flg/1 -> Detect Increase/1
  VINP_PsDoorSW_flg/1 -> Detect Increase1/1
  Detect Increase1/1 -> AND1/2
  Unit Delay2/1 -> AND1/1
  Constant1/1 -> Unit Delay2/1
  Constant2/1 -> Unit Delay3/1
  Unit Delay3/1 -> AND2/1
  Detect Increase2/1 -> AND2/2
  VINP_RLDoorSW_flg/1 -> Detect Increase2/1
  VINP_RRDoorSW_flg/1 -> Detect Increase3/1
  Detect Increase3/1 -> AND3/2
  Unit Delay4/1 -> AND3/1
  Constant3/1 -> Unit Delay4/1
  Constant4/1 -> Unit Delay5/1
  Unit Delay5/1 -> AND4/1
  Detect Increase4/1 -> AND4/2
  [VINP_TailgateSW_flg] -> Detect Increase4/1
  VINP_TailgateSW_flg/1 -> [VINP_TailgateSW_flg]
  [VINP_TailgateSW_flg] -> Chart/7(TailgateSW)
  AND/1 -> OR/1
  AND1/1 -> OR/2
  AND2/1 -> OR/3
  AND3/1 -> OR/4
  AND4/1 -> OR/5
  OR/1 -> [VBCM_DoorOpen_flg]
  [VBCM_DoorOpen_flg] -> Chart/5(DoorOpen)
  VINP_PDKeyAreaLockUnlock_enum/1 -> Chart/10(P_DKey_Area_LockUnlock)
  VINP_PDKeyAreaPS_enum/1 -> Chart/11(P_DKey_Area_PS)
  Chart/3(RoomLampTmr) -> Terminator/1  "VBCM_RoomLampTmr_s"
  KBCM_RmLpKeyInT_s/1 -> Chart/12(KBCM_RmLpKeyInT_s)  "2400"
  KBCM_RmLpKeyMissT_s/1 -> Chart/13(KBCM_RmLpKeyMissT_s)  "600"
  [task_time_s] -> Divide/2
  Divide/1 -> Chart/8(KBCM_RmLampKeep_min)
  task_time_s/1 -> [task_time_s]
  [task_time_s] -> Chart/1(task_time_s)

== system bcm/BCM/BCM/Tailgate ==
  VPMM_PwrSta_enum : Inport
  VINP_VehSpeed_kph : Inport  Port=2
  VBCM_BCMDoorLockSta_flg : Inport  Port=3
  VINP_TrunkHandleSwSG08_flg : Inport  Port=4
  Chart : Stateflow chart  TreatAsAtomicUnit=on
  VBCM_TrunkRel_flg : Outport
  VBCM_TailgateHDSW_flg : Outport  Port=2
  wires:
  VINP_VehSpeed_kph/1 -> Chart/2(VehSpeed)
  VBCM_BCMDoorLockSta_flg/1 -> Chart/3(DrLockSta)
  VINP_TrunkHandleSwSG08_flg/1 -> VBCM_TailgateHDSW_flg/1, Chart/4(TrunkHanSW)  "VBCM_TailgateHDSW_flg"
  Chart/1(TrunkRelease) -> VBCM_TrunkRel_flg/1  "VBCM_TrunkRel_flg"
  VPMM_PwrSta_enum/1 -> Chart/1(PwrSta)

== system bcm/BCM/BCM/Verify ==
  VINP_FlashAntitheft_enum : Inport
  Constant1 : Constant  Value=ENUM_ANTITHEFT_DISARM
  Constant10 : Constant  Value=ENUM_ANTITHEFT_WAIT
  Constant11 : Constant  Value=ENUM_ANTITHEFT_ALARM
  Constant9 : Constant  Value=ENUM_ANTITHEFT_ARM
  Equal1 : RelationalOperator  Operator=~=  OutDataTypeStr=boolean  RndMeth=Simplest
  Equal2 : RelationalOperator  Operator=~=  OutDataTypeStr=boolean  RndMeth=Simplest
  Equal3 : RelationalOperator  Operator=~=  OutDataTypeStr=boolean  RndMeth=Simplest
  Logical Operator : Logic  Inputs=3  AllPortsSameDT=off  OutDataTypeStr=boolean
  Switch : Switch  Criteria=u2 > Threshold
  VBCM_FlashAntitheft_enum : Outport
  wires:
  Constant9/1 -> Equal1/2
  VINP_FlashAntitheft_enum/1 -> [VINP_FlashAntitheft_enum]
  [VINP_FlashAntitheft_enum] -> Equal2/1
  [VINP_FlashAntitheft_enum] -> Equal1/1
  Constant11/1 -> Equal3/2
  Constant10/1 -> Equal2/2
  [VINP_FlashAntitheft_enum] -> Equal3/1
  Switch/1 -> VBCM_FlashAntitheft_enum/1
  Logical Operator/1 -> Switch/2
  Constant1/1 -> Switch/1
  [VINP_FlashAntitheft_enum] -> Switch/3
  Equal1/1 -> Logical Operator/1
  Equal2/1 -> Logical Operator/2
  Equal3/1 -> Logical Operator/3

== system bcm/BCM/BCM/WasherWiper ==
  VINP_CSWFWasSWSta_enum : Inport
  VINP_CSWFWipSWSta_enum : Inport  Port=2
  VINP_RLSRainSnrWiperCmd_enum : Inport  Port=3
  VINP_FWiperAS_flg : Inport  Port=4
  VINP_CSWRWipIntSwSta_enum : Inport  Port=5
  VINP_RWiperAS_flg : Inport  Port=6
  VINP_CSWRWasSWSta_enum : Inport  Port=7
  VPMM_PwrSta_enum : Inport  Port=8
  VINP_IVIWIMAINSW_flg : Inport  Port=9
  VINP_CANMsgValidIVI2_flg : Inport  Port=10
  VINP_RWiperProtection_flg : Inport  Port=11
  VINP_FWiperProtection_flg : Inport  Port=12
  VINP_FlashWiperFixMode : Inport  Port=13
  BCMInitial : Inport  Port=14
  Chart : Stateflow chart  TreatAsAtomicUnit=on
  Switch : Switch  Criteria=u2 > Threshold
  Switch1 : Switch  Criteria=u2 > Threshold
  Unit Delay : UnitDelay  SampleTime=-1  HasFrameUpgradeWarning=on
  VBCM_FrWiperL_flg : Outport
  VBCM_FrWiperH_flg : Outport  Port=2
  VBCM_RrWiper_flg : Outport  Port=3
  VBCM_WasherCtrl_enum : Outport  Port=4
  VBCM_WiperFixMode_flg : Outport  Port=5
  wires:
  VINP_FWiperProtection_flg/1 -> Chart/10(VINP_FWiperProtection_flg)
  VINP_RWiperProtection_flg/1 -> Chart/9(VINP_RWiperProtection_flg)
  Chart/1(FWiperL) -> VBCM_FrWiperL_flg/1  "VBCM_FrWiperL_flg"
  Chart/2(FWiperH) -> VBCM_FrWiperH_flg/1  "VBCM_FrWiperH_flg"
  VINP_RWiperAS_flg/1 -> Chart/6(RWiperAS)
  VINP_FWiperAS_flg/1 -> Chart/4(FWiperAS)
  VINP_CSWFWipSWSta_enum/1 -> Chart/2(CSW_FWipSw_Sta)
  VPMM_PwrSta_enum/1 -> Chart/8(PwrSta)
  VINP_CSWRWasSWSta_enum/1 -> Chart/7(CSW_RWasSW_Sta)
  VINP_CSWFWasSWSta_enum/1 -> Chart/1(CSW_FWasSw_Sta)
  Chart/3(RWiper) -> VBCM_RrWiper_flg/1  "VBCM_RrWiper_flg"
  VINP_RLSRainSnrWiperCmd_enum/1 -> Chart/3(RLS_RainSnrWiperCmd)
  Chart/4(WasherControl) -> VBCM_WasherCtrl_enum/1  "VBCM_WasherCtrl_enum"
  VINP_CSWRWipIntSwSta_enum/1 -> Chart/5(CSW_RWipIntSw_Sta)
  VINP_IVIWIMAINSW_flg/1 -> Switch/1
  VINP_CANMsgValidIVI2_flg/1 -> Switch/2  "VINP_CANMsgValidIVI2_flg"
  Unit Delay/1 -> Switch/3
  BCMInitial/1 -> Switch1/2
  VINP_FlashWiperFixMode/1 -> Switch1/3
  Switch1/1 -> VBCM_WiperFixMode_flg/1, Unit Delay/1  "VBCM_WiperFixMode_flg"
  Switch/1 -> Switch1/1

== system bcm/BCM/BCM/APM_Door/DoorAPM ==
  task_time_s : Inport
  DoorSW_flg : Inport  Port=2
  ControlCommand_pct : Inport  Port=3
  ValWdwOpened_pct : Inport  Port=4
  APMDoorControlSta_flg : Inport  Port=5
  WaitAPMPwr_K : Inport  Port=6
  DrOpenWdwOT_s : Inport  Port=7
  DrOpenWdwReady_s : Inport  Port=8
  KBCM_WdwManualDetT_K : Inport  Port=9
  CANMsgValidIVI2 : Inport  Port=10
  CANMsgValidGWZoneDR1 : Inport  Port=11
  CANMsgValidGWZoneFR1 : Inport  Port=12
  KBCM_DrAPMRetryTimes_cnt : Inport  Port=13
  Compare To Constant12 : simulink/Logic and Bit Operations/Compare To Constant  relop=>=  const=126  OutDataTypeStr=boolean
  Data Type Conversion{,1,4,8} (4 alike) : DataTypeConversion  OutDataTypeStr=uint8
  Data Type Conversion2 : DataTypeConversion  OutDataTypeStr=boolean
  Divide : Product  Inputs=*/
  Divide1 : Product  Inputs=*/
  Equal : RelationalOperator  OutDataTypeStr=boolean  RndMeth=Simplest
  Logical Operator : Logic  Operator=NOT  AllPortsSameDT=off  OutDataTypeStr=boolean
  Switch : Switch  Criteria=u2 ~= 0
  Timer : hcu_lib/Basic_Blocks/Timer
  Unit Delay : UnitDelay  SampleTime=-1  HasFrameUpgradeWarning=on
  Unit Delay9 : UnitDelay  SampleTime=-1  HasFrameUpgradeWarning=on
  window : Stateflow chart  TreatAsAtomicUnit=on
      settings: PortSchema="{\"entries\":[{\"content\":{\"sides\":[{\"content\":{\"connectorIds\":[\"In1\",\"In6\",\"In2\",\"In5\",\"In4\",\"In3\",\"In7\",\"In8\",\"In9\",\"In10\",\"In11\"]},\"type\":\"ConnectorPlacement.EquallySpacedRectSide\",\"uuid\":\"d6b3deb8-ac04-4a5e-8f43-f0925f49394b\"},{\"content\":{\"connectorIds\":[\"Out1\"],\"side\":\"RIGHT\"},\"type\":\"ConnectorPlacement.EquallySpacedRectSide\",\"uuid\":\"aa7d2074-5c17-49a8-96c4-41ae3a8edd6e\"},{\"content\":{\"side\":\"TOP\"},\"type\":\"ConnectorPlacement.EquallySpacedRectSide\",\"uuid\":\"a289e248-55db-4799-9cc5-9ff36bce4275\"}]},\"type\":\"ConnectorPlacement.EquallySpacedConnector\",\"uuid\":\"319072de-6de5-41b6-a853-dccc1445f214\"}],\"packageUris\":[\"http://schema.mathworks.com/mf0/Connector/R2020b\"],\"version\":\"1.0\"}"
  CtrlCmd_pct : Outport
  CtrlCmdReady_flg : Outport  Port=2
  wires:
  Data Type Conversion2/1 -> window/5(CtrlCmd_Ready)
  KBCM_DrAPMRetryTimes_cnt/1 -> window/11(KBCM_DrAPMRetryTimes_cnt)
  CANMsgValidGWZoneFR1/1 -> window/10(CANMsgValidGWZoneFR1)
  CANMsgValidGWZoneDR1/1 -> window/9(CANMsgValidGWZoneDR1)
  ControlCommand_pct/1 -> Switch/1
  Unit Delay/1 -> Switch/3
  Switch/1 -> Unit Delay/1, Data Type Conversion8/1
  CANMsgValidIVI2/1 -> Switch/2
  Divide1/1 -> Data Type Conversion1/1
  Data Type Conversion1/1 -> window/8(KBCM_WdwManualDetT_K)
  KBCM_WdwManualDetT_K/1 -> Divide1/1
  [task_time_s] -> Divide1/2
  [DrOpenWdwReady_s] -> Equal/2
  [DrOpenWdwReady_s] -> Timer/4
  DrOpenWdwReady_s/1 -> [DrOpenWdwReady_s]
  DrOpenWdwOT_s/1 -> Divide/1
  [task_time_s] -> Divide/2
  Divide/1 -> Data Type Conversion4/1
  WaitAPMPwr_K/1 -> window/3(WaitAPMPwr_K)
  APMDoorControlSta_flg/1 -> window/4(APMDoorControlSta)
  task_time_s/1 -> [task_time_s]
  Unit Delay9/1 -> Data Type Conversion2/1
  ValWdwOpened_pct/1 -> Data Type Conversion/1
  [task_time_s] -> Timer/3
  [CtrlCmdReady_flg] -> Unit Delay9/1
  Logical Operator/1 -> Timer/2
  Data Type Conversion/1 -> window/2(Val_Wdw_Opened)
  DoorSW_flg/1 -> window/1(DoorSW)
  Data Type Conversion4/1 -> window/7(DrOpenWdwOT_K)
  Compare To Constant12/1 -> Timer/1, Logical Operator/1
  window/1(CtrlCmd) -> CtrlCmd_pct/1, Compare To Constant12/1
  Timer/1 -> Equal/1
  Data Type Conversion8/1 -> window/6(ControlCommand)
  Equal/1 -> [CtrlCmdReady_flg], CtrlCmdReady_flg/1

== system bcm/BCM/BCM/AntiTheft/Antitheft__override ==
  In1 : Inport
  Constant : Constant  Value=KBCM_Antitheft_enum_ovrdflg
  Constant1 : Constant  Value=KBCM_Antitheft_enum_ovrdval
  Switch : Switch  Criteria=u2 > Threshold
  Out1 : Outport
  wires:
  Constant/1 -> Switch/2
  Switch/1 -> Out1/1
  In1/1 -> Switch/3
  Constant1/1 -> Switch/1

== system bcm/BCM/BCM/ExteriorLight/HeadLampErrorHanding ==
  VINP_HeadLampSW_enum : Inport
  VINP_CANMsgValidIVI2_flg : Inport  Port=2
  Add : Sum
  Compare To Constant : simulink/Logic and Bit Operations/Compare To Constant  relop=>=  const=1000  OutDataTypeStr=boolean
  Constant : Constant
  Constant1 : Constant  Value=0
  Constant2 : Constant  Value=0
  Constant3 : Constant  Value=0
  Saturation : Saturate  UpperLimit=1000  LowerLimit=0
  Switch{,1..3} (4 alike) : Switch  Criteria=u2 > Threshold
  Unit Delay : UnitDelay  SampleTime=-1  HasFrameUpgradeWarning=on
  Unit Delay1 : UnitDelay  SampleTime=-1  HasFrameUpgradeWarning=on
  VBCM_HeadLampSW_enum : Outport
  wires:
  VINP_CANMsgValidIVI2_flg/1 -> Switch2/2, Switch/2
  Switch2/1 -> Switch3/3, Unit Delay/1
  Unit Delay/1 -> Switch2/3
  VINP_HeadLampSW_enum/1 -> Switch2/1
  Switch/1 -> Switch1/2, Add/2
  Unit Delay1/1 -> Add/1
  Add/1 -> Switch1/1
  Constant/1 -> Switch/3
  Constant1/1 -> Switch/1
  Constant2/1 -> Switch1/3
  Constant3/1 -> Switch3/1
  Switch3/1 -> VBCM_HeadLampSW_enum/1
  Compare To Constant/1 -> Switch3/2
  Saturation/1 -> Unit Delay1/1, Compare To Constant/1
  Switch1/1 -> Saturation/1
